simulink model "rotpentemplate"  (R2021b)
settings: Solver=ode45  StartTime=0.0  StopTime=30  RelTol=1e-3  EnableMultiTasking=on
undefined symbols (not defined in the file): adingain, adinoffs, daoutgain, daoutoffs, ekfInputParameters, h, sampleTime
libraries: sharedTrackingLibrary x1
settings Model: Creator=rbabuska  LastModifiedBy=tsderksen
settings SolverCC: AlgebraicLoopSolver=TrustRegion
settings DataIOCC: LimitDataPoints=on  SaveFormat=Array  ReturnWorkspaceOutputs=off  SignalLoggingName=sigsOut
settings OptimizationCC: BooleanDataType=off  ExpressionDepthLimit=2147483647  InitFltsAndDblsToZero=on  LifeSpan=inf
settings DebuggingCC: SaveWithParameterizedLinksMsg=none  SignalResolutionControl=TryResolveAllWithWarning  MultiTaskDSMMsg=warning  MultiTaskCondExecSysMsg=none  AllowSymbolicDim=off  StateNameClashWarn=warning  SFUnexpectedBacktrackingDiag=warning  SFNoUnconditionalDefaultTransitionDiag=warning  SFExecutionAtInitializationDiag=none  SFMachineParentedDataDiag=warning  ArithmeticOperatorsInVariantConditions=warning
settings HardwareCC: ProdBitPerPointer=32  ProdBitPerSizeT=32  ProdBitPerPtrDiffT=32  ProdLargestAtomicFloat=None  ProdIntDivRoundTo=Undefined  ProdEndianess=Unspecified  ProdWordSize=32  ProdHWDeviceType=32-bit Generic  TargetUnknown=on
settings ModelReferenceCC: PropagateSignalLabelsOutOfModel=off
settings SFSimCC: SimUseLocalCustomCode=off  CustomCodeUndefinedFunction=UseInterfaceOnly
settings RTWCC: RTWUseLocalCustomCode=off
settings CodeAppCC: StateflowObjectComments=on
settings GRTTargetCC: TargetFcnLib=ansi_tfl_tmw.mat  TargetLangStandard=C89/C90 (ANSI)  CombineOutputUpdateFcns=off  GRTInterface=on
settings ConfigComp: CovMetricSettings=dw  CovSaveCumulativeToWorkspaceVar=on  CovSaveSingleToWorkspaceVar=on  CovExternalEMLEnable=off

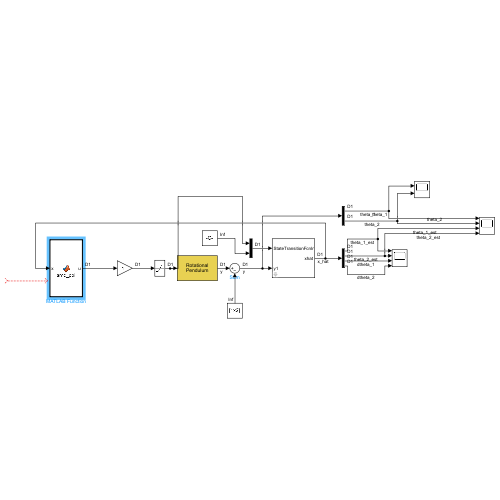
[thumbnail: Simulink's stored preview of the top-level diagram]
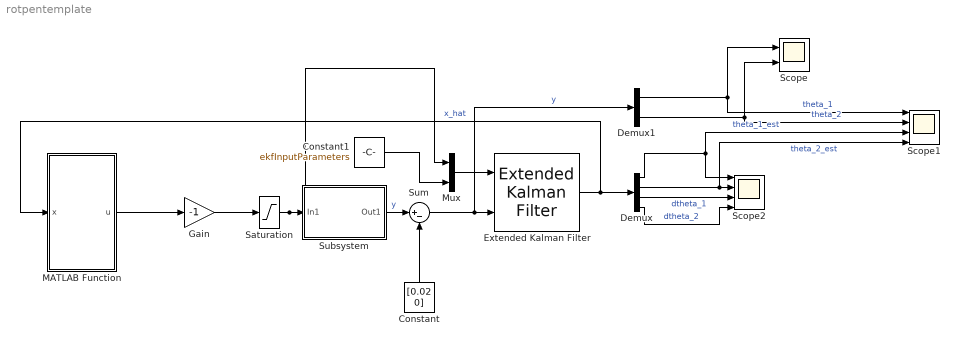
== system rotpentemplate ==
  Constant : Constant  Value=[0.02 0]
  Constant1 : Constant  Value=ekfInputParameters
  Demux : Demux
  Demux1 : Demux  Outputs=2
  Extended Kalman Filter : sharedTrackingLibrary/Extended Kalman Filter  StateTransitionFcn=rotpendulumEkfStateTransition  HasStateTransitionJacobianFcn=off  HasAdditiveProcessNoise=Additive  ProcessNoise=diag([1e-4 1e-4 1e-4 1e-3])  HasTimeVaryingProcessNoise=off  HasStateTransitionFcnExtraArgument=1  InitialState=x0  InitialStateCovariance=P0_ekf  MeasurementFcn1=rotpendulumEkfMeasurement  HasMeasurementJacobianFcn1=off  HasMeasurementEnablePort1=off  HasAdditiveMeasurementNoise1=Additive  MeasurementNoise1=R_ekf  HasTimeVaryingMeasurementNoise1=off  HasMeasurementFcnExtraArgument1=0  MeasurementFcn2=myMeasurementFcn  HasMeasurementJacobianFcn2=off  HasMeasurementEnablePort2=off  HasAdditiveMeasurementNoise2=Additive  MeasurementNoise2=1  HasTimeVaryingMeasurementNoise2=off  HasMeasurementFcnExtraArgument2=0  MeasurementFcn3=myMeasurementFcn  HasMeasurementJacobianFcn3=off  HasMeasurementEnablePort3=off  HasAdditiveMeasurementNoise3=Additive  MeasurementNoise3=1  HasTimeVaryingMeasurementNoise3=off  HasMeasurementFcnExtraArgument3=0  MeasurementFcn4=myMeasurementFcn  HasMeasurementJacobianFcn4=off  HasMeasurementEnablePort4=off  HasAdditiveMeasurementNoise4=Additive  MeasurementNoise4=1  HasTimeVaryingMeasurementNoise4=off  HasMeasurementFcnExtraArgument4=0  MeasurementFcn5=myMeasurementFcn  HasMeasurementJacobianFcn5=off  HasMeasurementEnablePort5=off  HasAdditiveMeasurementNoise5=Additive  MeasurementNoise5=1  HasTimeVaryingMeasurementNoise5=off  HasMeasurementFcnExtraArgument5=0  EnableMultirate=off  StateTransitionFcnSampleTime=1  MeasurementFcn1SampleTime=1  MeasurementFcn2SampleTime=1  MeasurementFcn3SampleTime=1  MeasurementFcn4SampleTime=1  MeasurementFcn5SampleTime=1  UseCurrentEstimator=on  OutputStateCovariance=off  DataType=double  SampleTime=sampleTime  NumberOfMeasurements=1
      settings: SourceProductBaseCode=AE,PW,CT,DR,TF,ID,LP,NV,AR,RO,RR,UV,VE
  Gain : Gain  Gain=-1
  MATLAB Function : MATLAB Function  TreatAsAtomicUnit=on
  Mux : Mux  Inputs=2
  Saturation : Saturate  UpperLimit=1  LowerLimit=-1
  Scope : Scope  NumInputPorts=2
  Scope1 : Scope  NumInputPorts=4
  Scope2 : Scope  NumInputPorts=4
  Subsystem : Subsystem
      mask Display: disp('Rotational\nPendulum')
  Sum : Sum  Inputs=|+-
  wires:
  Saturation/1 -> Mux/1, Subsystem/1(In1)
  Sum/1 -> Demux1/1, Extended Kalman Filter/2  "y"
  Mux/1 -> Extended Kalman Filter/1
  Constant1/1 -> Mux/2
  Extended Kalman Filter/1 -> MATLAB Function/1(x), Demux/1  "x_hat"
  Demux1/1 -> Scope1/1, Scope/1  "theta_1"
  Demux1/2 -> Scope/2, Scope1/2  "theta_2"
  Demux/1 -> Scope1/3, Scope2/1  "theta_1_est"
  Demux/2 -> Scope1/4, Scope2/2  "theta_2_est"
  Demux/3 -> Scope2/3  "dtheta_1"
  Demux/4 -> Scope2/4  "dtheta_2"
  MATLAB Function/1(u) -> Gain/1
  Gain/1 -> Saturation/1
  ? -> ?
  Subsystem/1(Out1) -> Sum/1  "y"
  Constant/1 -> Sum/2

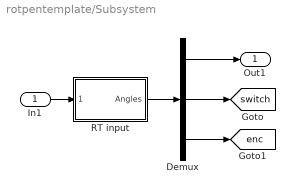
== system rotpentemplate/Subsystem ==
  In1 : Inport
  Demux : Demux  Outputs=[2 4 1]
  RT input : Subsystem  mask{Ts=h, channels=[6 7]}
      mask prompts: Ts "Sample time [s]:"; channels "Channels to read (e.g., [6 7])"
      mask init:
      | hwinit;
      | 
      | % initialize FPGA
      | fugihandle = fugiboard('Open', 'Pendulum1');
      | fugihandle.WatchdogTimeout = 0.5;
      | fugiboard('SetParams', fugihandle);
      | fugiboard('Write', fugihandle, 0, 0, 0, 0);  % dummy write to sync interface board
      | fugiboard('Write', fugihandle, 5, 1, 0, 0);  % reset position, activate relay
      | data = fugiboard('Read', fugihandle);        % get version info from FPGA
      | % model = bitshift(data(1), -5); 
      | % version = bitand(data(1), 31);
      | % disp(sprintf('FPGA setup %d, version %d', model, version)); % for the B&P it should say 1 1, or else there is a problem
      | fugiboard('Write', fugihandle, 0, 1, 0, 0);  % end reset
      | pause(0.1);                         % give relay some time to respond
      mask Display: disp('Rotational\nPendulum')
  Out1 : Outport
  tag scope: enc=global, switch=global
  wires:
  RT input/1(Angles) -> Demux/1
  Demux/1 -> Out1/1
  Demux/2 -> [switch]
  Demux/3 -> [enc]
  In1/1 -> RT input/1(Motors)

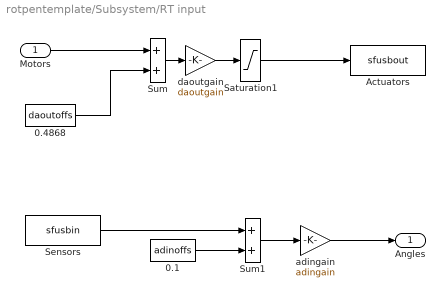
== system rotpentemplate/Subsystem/RT input ==
  Motors : Inport
  0.1 : Constant  Value=adinoffs
  0.4868 : Constant  Value=daoutoffs
  Actuators : S-Function  FunctionName=sfusbout  Parameters=Ts, fugihandle  SFunctionDeploymentMode=off  EnableBusSupport=off
  Saturation1 : Saturate  UpperLimit=10  LowerLimit=-10
  Sensors : S-Function  FunctionName=sfusbin  Parameters=Ts, fugihandle, channels  SFunctionDeploymentMode=off  EnableBusSupport=off
  Sum : Sum  InputSameDT=on  SaturateOnIntegerOverflow=on  OutDataTypeStr=Inherit: Same as first input
  Sum1 : Sum  InputSameDT=on  SaturateOnIntegerOverflow=on  OutDataTypeStr=Inherit: Same as first input
  adingain : Gain  Gain=adingain  SaturateOnIntegerOverflow=on  OutDataTypeStr=Inherit: Same as input  ParamDataTypeStr=Inherit: Same as input
  daoutgain : Gain  Gain=daoutgain  SaturateOnIntegerOverflow=on  OutDataTypeStr=Inherit: Same as input  ParamDataTypeStr=Inherit: Same as input
  Angles : Outport
  wires:
  Sum/1 -> daoutgain/1
  0.4868/1 -> Sum/2
  Motors/1 -> Sum/1
  Sum1/1 -> adingain/1
  0.1/1 -> Sum1/2
  adingain/1 -> Angles/1
  Saturation1/1 -> Actuators/1
  daoutgain/1 -> Saturation1/1
  Sensors/1 -> Sum1/1

== matlab function rotpentemplate/MATLAB Function ==
  data: x input; u output
function u = smc_ppi(x)            %#codegen
    x = x(:);                      % force 4x1 column (kills orientation error)

    % ---- parameters (must match your identified plant) ----
    pa=64.7915; pb1=3.2117e3; pc1=635.3865; pg1=430.5226; pu=2.2424e4;
    pb2=0.0670; pg2=112.0268; pc2=0.2491; psdelta2=0.1836;
    epsv1=0.05; epsv2=0.03; vs2=3.5;  l1=0.1; g=9.81;
    pc=(l1/g)*pg2;

    % ---- design constants ----
    c    = [19.9432; 27.7084; 0.3566; 1.5661];   % B'P sliding vector
    k    = 40;                     % switching gain   -- TUNE
    phi  = 1;                    % boundary layer   -- TUNE
    xref = [pi; pi; 0; 0];

    % ---- sliding variable (with angle wrapping) ----
    e    = x - xref;
    e(1) = mod(e(1)+pi,2*pi)-pi;
    e(2) = mod(e(2)+pi,2*pi)-pi;
    s    = c.'*e;

    % ---- inlined drift f0 = f(x,0) ----
    th1=x(1); th2=x(2); d1=x(3); d2=x(4);
    c2=cos(th2); s2=sin(th2);
    M11=pa+1+2*pc*c2; M12=1+pc*c2; M22=1; detM=M11*M22-M12*M12;
    Cq1=-pc*s2*(2*d1*d2+d2^2);
    Cq2= pc*s2*d1^2;
    F1 = pb1*d1 + pc1*tanh(d1/epsv1);
    strib = pc2 + psdelta2*exp(-(d2/vs2)^2);
    F2 = pb2*d2 + strib*tanh(d2/epsv2);
    G1 = -pg1*sin(th1) - pg2*sin(th1+th2);
    G2 = -pg2*sin(th1+th2);
    r1 = -Cq1 - F1 - G1;           % u = 0 here
    r2 = -Cq2 - F2 - G2;
    dd1 = ( M22*r1 - M12*r2)/detM;
    dd2 = (-M12*r1 + M11*r2)/detM;
    f0  = [d1; d2; dd1; dd2];

    % ---- SMC law ----
    cg  = (pu/detM)*( c(3) - c(4)*M12 );   % c'*g(x)
    ueq = -(c.'*f0)/cg;
    usw = -(k/cg)*max(min(s/phi,1),-1);
    u   = max(min(ueq + usw, 1), -1);      % scalar, saturated
end
